simulink model "trajectory"  (R2019b)
settings: Solver=VariableStepAuto  StartTime=0.0  StopTime=10.0  RelTol=1e-3
values from neighbouring files (symbols this model uses):
  A = 0.005    [Railgun.m]
  Cd = 0.1    [Railgun.m]
  g = 9.81    [Railgun.m]
  Massofprojectile = 0.1    [Railgun.m]
  Rho = 1.225    [Railgun.m]
settings Model: Creator=keato  LastModifiedBy=keato

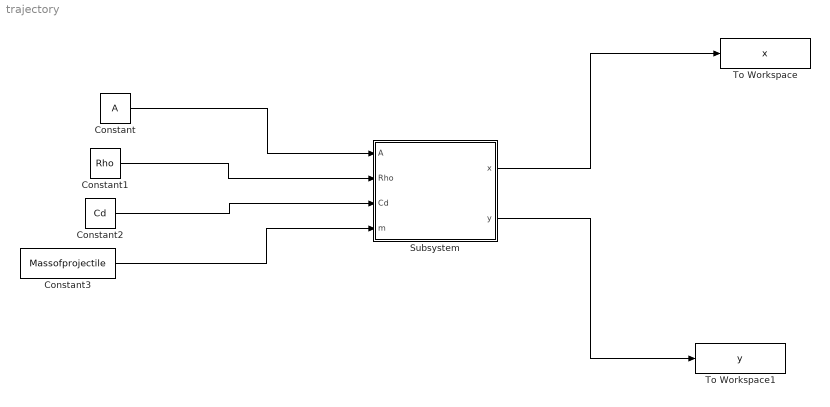
== system trajectory ==
  Constant : Constant  Value=A
  Constant1 : Constant  Value=Rho
  Constant2 : Constant  Value=Cd
  Constant3 : Constant  Value=Massofprojectile
  Subsystem : Subsystem
  To Workspace : ToWorkspace  VariableName=x  SaveFormat=Timeseries  SampleTime=-1
  To Workspace1 : ToWorkspace  VariableName=y  SaveFormat=Timeseries  SampleTime=-1
  wires:
  Constant/1 -> Subsystem/1(A)
  Constant1/1 -> Subsystem/2(Rho)
  Constant2/1 -> Subsystem/3(Cd)
  Constant3/1 -> Subsystem/4(m)
  Subsystem/1(x) -> To Workspace/1
  Subsystem/2(y) -> To Workspace1/1

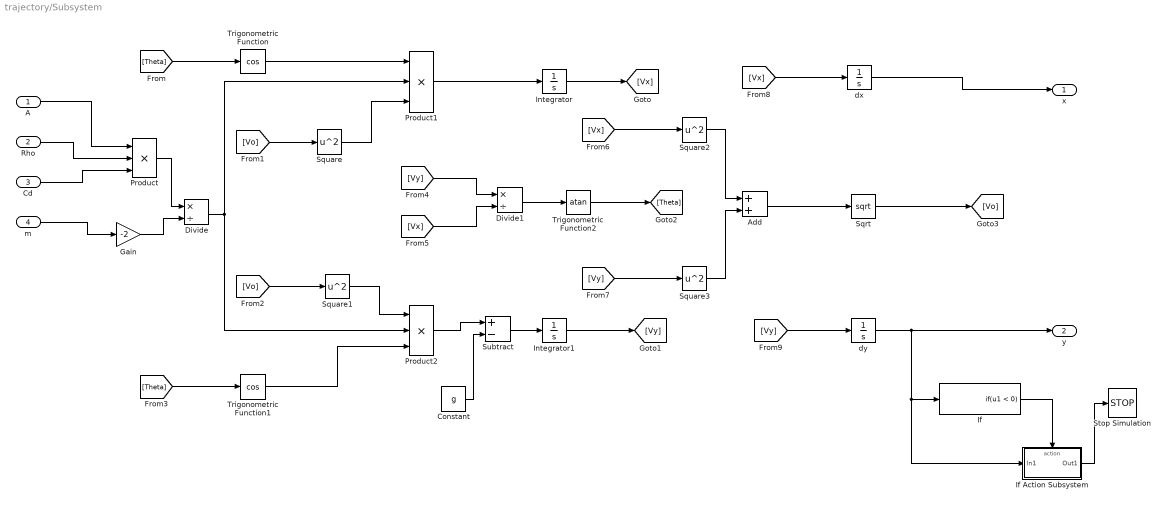
== system trajectory/Subsystem ==
  A : Inport
  Rho : Inport  Port=2
  Cd : Inport  Port=3
  m : Inport  Port=4
  Add : Sum
  Constant : Constant  Value=g
  Divide : Product  Inputs=*/
  Divide1 : Product  Inputs=*/
  Gain : Gain  Gain=-2
  If : If  IfExpression=u1 < 0  ShowElse=off
  If Action Subsystem : Subsystem  TreatAsAtomicUnit=on
  Integrator : Integrator
  Integrator1 : Integrator
  Product : Product  Inputs=3
  Product1 : Product  Inputs=3
  Product2 : Product  Inputs=3
  Sqrt : Sqrt  SaturateOnIntegerOverflow=on
  Square{,1..3} (4 alike) : Math  Operator=square  SignedPower=off  SaturateOnIntegerOverflow=on
  Stop Simulation : Stop
  Subtract : Sum  Inputs=+-
  Trigonometric Function : Trigonometry  Operator=cos
  Trigonometric Function1 : Trigonometry  Operator=cos
  Trigonometric Function2 : Trigonometry  Operator=atan
  dx : Integrator
  dy : Integrator
  x : Outport
  y : Outport  Port=2
  wires:
  Square2/1 -> Add/1
  Subtract/1 -> Integrator1/1
  Product/1 -> Divide/1
  Product1/1 -> Integrator/1
  Trigonometric Function1/1 -> Product2/3
  dx/1 -> x/1
  [Vx] -> Square2/1
  Constant/1 -> Subtract/2
  [Vx] -> dx/1
  Divide/1 -> Product2/2, Product1/2
  m/1 -> Gain/1
  Trigonometric Function/1 -> Product1/1
  Square/1 -> Product1/3
  [Vy] -> dy/1
  Integrator1/1 -> [Vy]
  [Vy] -> Square3/1
  Integrator/1 -> [Vx]
  Trigonometric Function2/1 -> [Theta]
  Add/1 -> Sqrt/1
  dy/1 -> y/1, If Action Subsystem/1(In1), If/1
  [Vy] -> Divide1/1
  [Vx] -> Divide1/2
  [Vo] -> Square1/1
  Square3/1 -> Add/2
  Divide1/1 -> Trigonometric Function2/1
  [Theta] -> Trigonometric Function1/1
  [Theta] -> Trigonometric Function/1
  Sqrt/1 -> [Vo]
  If/1 -> If Action Subsystem/Action
  If Action Subsystem/1(Out1) -> Stop Simulation/1
  Cd/1 -> Product/3
  A/1 -> Product/1
  Product2/1 -> Subtract/1
  Gain/1 -> Divide/2
  Rho/1 -> Product/2
  [Vo] -> Square/1
  Square1/1 -> Product2/1

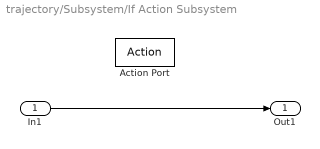
== system trajectory/Subsystem/If Action Subsystem ==
  In1 : Inport
  Action Port : ActionPort  ActionPortLabel=if(u1 < 0)
  Out1 : Outport
  wires:
  In1/1 -> Out1/1
